simulink model "motor_pid"  (R2018a)
settings: Solver=ode45  StartTime=0.0  StopTime=1  FixedStep=1e-4  RelTol=1e-4
InitFcn:
  | Tw=0.01;     %Ancho de Ventana
  | ppv=20;      %Pulsos por vuelta
  | Ts=1e-4;     %Tiempo de muestreo
  | 
  | Kp=0.001;
  | Kd=0.02;
  | Ki=0.4;
  | h=Tw;
  | N=100;
settings Model: Creator=Martin  LastModifiedBy=Alan
settings CodeAppCC: StateflowObjectComments=on

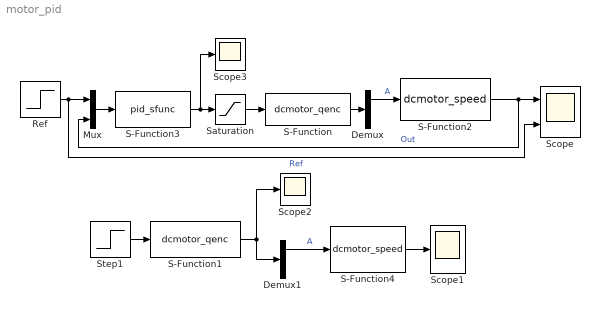
== system motor_pid ==
  Demux : Demux  Outputs=2
  Demux1 : Demux  Outputs=2
  Mux : Mux  Inputs=2
  Ref : Step  Time=0.2  After=4200  SampleTime=Ts
  S-Function : S-Function  FunctionName=dcmotor_qenc  Parameters=ppv  SFunctionDeploymentMode=off  EnableBusSupport=off
  S-Function1 : S-Function  FunctionName=dcmotor_qenc  Parameters=ppv  SFunctionDeploymentMode=off  EnableBusSupport=off
  S-Function2 : S-Function  FunctionName=dcmotor_speed  Parameters=Ts,ppv,Tw  SFunctionDeploymentMode=off  EnableBusSupport=off
  S-Function3 : S-Function  FunctionName=pid_sfunc  Parameters=Kp,Kd,Ki,h,N  SFunctionDeploymentMode=off  EnableBusSupport=off
  S-Function4 : S-Function  FunctionName=dcmotor_speed  Parameters=Ts,ppv,Tw  SFunctionDeploymentMode=off  EnableBusSupport=off
  Saturation : Saturate  UpperLimit=30  LowerLimit=-30
  Scope : Scope  NumInputPorts=2
  Scope1 : Scope
  Scope2 : Scope
  Scope3 : Scope
  Step1 : Step  Time=0.5  After=12  SampleTime=Ts
  wires:
  Ref/1 -> Mux/1, Scope/2  "Ref"
  S-Function/1 -> Demux/1
  Demux/1 -> S-Function2/1  "A"
  S-Function2/1 -> Scope/1, Mux/2  "Out"
  Mux/1 -> S-Function3/1
  Saturation/1 -> S-Function/1
  S-Function3/1 -> Scope3/1, Saturation/1
  Demux1/1 -> S-Function4/1  "A"
  Step1/1 -> S-Function1/1
  S-Function1/1 -> Demux1/1, Scope2/1
  S-Function4/1 -> Scope1/1
